simulink model "Lab5_Discrete"  (R2020a)
settings: Solver=VariableStepAuto  StartTime=0.0  StopTime=2500  RelTol=1e-3
libraries: simulink x1
settings Model: Creator=mitch  LastModifiedBy=noah-

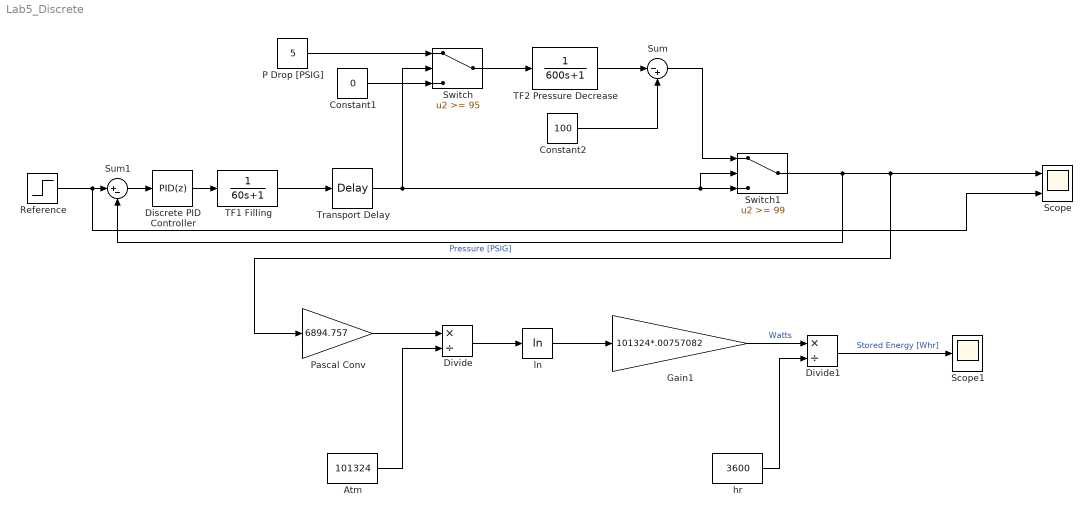
== system Lab5_Discrete ==
  Atm : Constant  Value=101324
  Constant1 : Constant  Value=0
  Constant2 : Constant  Value=100
  Discrete PID Controller : simulink/Continuous/PID Controller  Controller=PID  Form=Parallel  TimeDomain=Discrete-time  UseExternalTs=off  SampleTime=20  IntegratorMethod=Forward Euler  FilterMethod=Forward Euler  ControllerParametersSource=internal  P=0.0190248710112501  I=0.00190248710112501  D=0  UseFilter=on  N=100  TunerSelectOption=Transfer Function Based (PID Tuner App)  InitialConditionSource=internal  InitialConditionForIntegrator=0  InitialConditionForFilter=0  DifferentiatorICPrevScaledInput=0  ExternalReset=none  TrackingMode=off  Kt=1  LimitOutput=off  UpperSaturationLimit=inf  LowerSaturationLimit=-inf  LinearizeAsGain=off  AntiWindupMode=none  Kb=1  POutMin=[]  POutMax=[]  IOutMin=[]  IOutMax=[]  DOutMin=[]  DOutMax=[]  NOutMin=[]  NOutMax=[]  SumOutMin=[]  SumOutMax=[]  SaturationOutMin=[]  SaturationOutMax=[]  PParamMin=[]  PParamMax=[]  IParamMin=[]  IParamMax=[]  DParamMin=[]  DParamMax=[]  NParamMin=[]  NParamMax=[]  KbParamMin=[]  KbParamMax=[]  KtParamMin=[]  KtParamMax=[]  KbOutMin=[]  KbOutMax=[]  KtOutMin=[]  KtOutMax=[]  IntegratorOutMin=[]  IntegratorOutMax=[]  FilterOutMin=[]  FilterOutMax=[]  SumI1OutMin=[]  SumI1OutMax=[]  SumI2OutMin=[]  SumI2OutMax=[]  SumI3OutMin=[]  SumI3OutMax=[]  SumI4OutMin=[]  SumI4OutMax=[]  SumDOutMin=[]  SumDOutMax=[]  DifferentiatorOutMin=[]  DifferentiatorOutMax=[]  FilterDiffOutCoefMin=[]  FilterDiffOutCoefMax=[]  ReciprocalOutMin=[]  ReciprocalOutMax=[]  SumDenOutMin=[]  SumDenOutMax=[]  SumNumOutMin=[]  SumNumOutMax=[]  DivideOutMin=[]  DivideOutMax=[]  UdiffTsProdOutMin=[]  UdiffTsProdOutMax=[]  NTsProdOutMin=[]  NTsProdOutMax=[]  UintegralTsProdOutMin=[]  UintegralTsProdOutMax=[]  UngainTsProdOutMin=[]  UngainTsProdOutMax=[]  IntegratorContinuousStateAttributes=''  IntegratorStateMustResolveToSignalObject=off  IntegratorRTWStateStorageClass=Auto  FilterContinuousStateAttributes=''  FilterStateMustResolveToSignalObject=off  FilterRTWStateStorageClass=Auto  ParallelPVariant=InternalParameters  IdealPVariant=Disabled  IVariant=InternalParameters  DVariant=InternalParameters  IntegratorVariant=Discrete  SatVariant=Disabled  AWVariant=Passthrough  PCopyVariant=Disabled  TRVariant=Disabled  FdbkBlocksVariant=Forward  IdealPFdbkVariant=Disabled  SatFdbkVariant=Disabled  DerivativeFilterVariant=ForwardEulerFilter  NVariant=InternalParameters  NCopyVariant=Disabled  FilterICVariant=InternalICsFilter  IntegratorICVariant=InternalICs  ExternalResetVariant=Disabled  TRSumVariant=Passthrough  SumFdbkVariant=Disabled  SumVariant=Sum_PID  TsampFilterVariant=InternalTs  TsampNgainVariant=Passthrough  TsampIntegralVariant=Passthrough
  Divide : Product  Inputs=*/
  Divide1 : Product  Inputs=*/
  Gain1 : Gain  Gain=101324*.00757082
  P Drop [PSIG] : Constant  Value=5
  Pascal Conv : Gain  Gain=6894.757
  Reference : Step  Time=10  After=100  SampleTime=0
  Scope : Scope  NumInputPorts=2
  Scope1 : Scope
  Sum : Sum  Inputs=|-+
  Sum1 : Sum  Inputs=|+-
  Switch : Switch  Threshold=95
  Switch1 : Switch  Threshold=99
  TF1 Filling : TransferFcn  Denominator=[60 1]
  TF2 Pressure Decrease : TransferFcn  Denominator=[600 1]
  Transport Delay : TransportDelay
  hr : Constant  Value=3600
  ln : Math  Operator=log  SaturateOnIntegerOverflow=on
  wires:
  Constant2/1 -> Sum/2
  TF2 Pressure Decrease/1 -> Sum/1
  Pascal Conv/1 -> Divide/1
  Atm/1 -> Divide/2
  Divide/1 -> ln/1
  ln/1 -> Gain1/1
  Gain1/1 -> Divide1/1  "Watts"
  hr/1 -> Divide1/2
  TF1 Filling/1 -> Transport Delay/1
  P Drop [PSIG]/1 -> Switch/1
  Transport Delay/1 -> Switch/2, Switch1/2, Switch1/3
  Constant1/1 -> Switch/3
  Switch/1 -> TF2 Pressure Decrease/1
  Sum/1 -> Switch1/1
  Switch1/1 -> Sum1/2, Pascal Conv/1, Scope/1  "Pressure [PSIG]"
  Sum1/1 -> Discrete PID Controller/1
  Reference/1 -> Scope/2, Sum1/1
  Discrete PID Controller/1 -> TF1 Filling/1
  Divide1/1 -> Scope1/1  "Stored Energy [Whr]"
